simulink model "bpskRCdelayLG"  (Simulink 8.6)
settings: Solver=VariableStepAuto  StartTime=0.0  StopTime=10.0  RelTol=1e-3
values from neighbouring files (symbols this model uses):
  delay = .75    (= 0.75)    [lab02.m]    (also in setup.m = 0.5)
  filterspan = 4    [lab02.m]    (also in setup.m)
  outputSamples = 8    [lab02.m]    (also in setup.m)
  rolloff = .5    (= 0.5)    [lab02.m]    (also in setup.m)
  sampleTime = 1/R    (= 1.0272213662e-05)    [lab02.m]    (also in setup.m)
libraries: commdigbbndpm3 x2, commfilt2 x2, commchan3 x1, commsink2 x1, commsync2 x1, dspsigops x1
settings Model: Creator=tim  LastModifiedBy=tim
settings DataIOCC: SaveFormat=Dataset  SignalLoggingSaveFormat=Dataset
settings OptimizationCC: ExpressionDepthLimit=128
settings DebuggingCC: UnderspecifiedInitializationDetection=Simplified  MergeDetectMultiDrivingBlocksExec=error  SolverPrmCheckMsg=none  FcnCallInpInsideContextMsg=EnableAllAsError  StateNameClashWarn=none
settings HardwareCC: ProdBitPerPointer=64  ProdLargestAtomicFloat=Float  ProdIntDivRoundTo=Zero  ProdEndianess=LittleEndian  ProdWordSize=64  ProdHWDeviceType=Intel->x86-64 (Windows64)
settings GRTTargetCC: GeneratePreprocessorConditionals=Use local settings  CombineOutputUpdateFcns=on  GRTInterface=off
settings ConfigComp: CovModelRefEnable=off

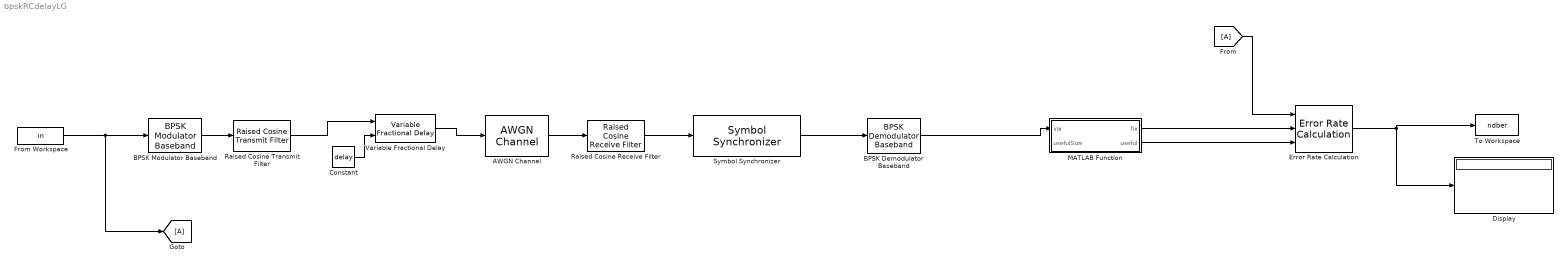
== system bpskRCdelayLG ==
  AWGN Channel : commchan3/AWGN Channel  InputProcessing=Columns as channels (frame based)  seed=67  noiseMode="Signal to noise ratio  (SNR)"  EbNodB=snr  EsNodB=10  SNRdB=snr  bitsPerSym=1  Ps=1  Tsym=1  variance=1
  BPSK Demodulator Baseband : commdigbbndpm3/BPSK Demodulator Baseband  Ph=0  DecType=Hard decision  VarSource=Dialog  Variance=1  outDtype=Inherit via internal rule  derotateFactorWordLen=16
  BPSK Modulator Baseband : commdigbbndpm3/BPSK Modulator Baseband  Ph=0  outDtype=double  outWordLen=16  outUDDataType=sfix(16)  outFracLenMode=Best precision  outFracLen=15
  Constant : Constant  Value=delay
  Display : Display
  Error Rate Calculation : commsink2/Error Rate Calculation  N=0  st_delay=0  cp_mode=Select samples from port  subframe=[]  PMode=Port  WsName=ErrorVec  RsMode2=off  stop=on  numErr=maxErrors  maxBits=maxBits
  From Workspace : FromWorkspace  VariableName=in  SampleTime=sampleTime  Interpolate=off  OutputAfterFinalValue=Cyclic repetition
  MATLAB Function : MATLAB Function  TreatAsAtomicUnit=on
  Raised Cosine Receive Filter : commfilt2/Raised Cosine Receive Filter  filtType=Square root  N=8  filtSpan=4  currentFiltSpan=4  D=(4)/2  R=.5  sampMode=Mute  saveAsFlag=0  rateMode=Downsampling  downFactor=1  downOffset=0  framing=Enforce single-rate processing  InputProcessing=Columns as channels (frame based)  checkGain=Normalized  filterGain=1  checkCoeff=off  variableName=rcRxFilt  launchFVT=on  roundingMode=Floor  overflowMode=off
  Raised Cosine Transmit Filter : commfilt2/Raised Cosine Transmit Filter  filtType=Square root  filtSpan=filterspan  currentFiltSpan=filterspan  D=(filterspan)/2  R=rolloff  sampMode=Mute  saveAsFlag=0  N=outputSamples  framing=Enforce single-rate processing  InputProcessing=Columns as channels (frame based)  checkGain=Normalized  filterGain=linearAmp  checkCoeff=off  variableName=rcTxFilt  launchFVT=on  roundingMode=Floor  overflowMode=off
  Symbol Synchronizer : commsync2/Symbol Synchronizer  TimingErrorDetector=Early-Late (non-data-aided)  SamplesPerSymbol=8  DampingFactor=1  NormalizedLoopBandwidth=.001  DetectorGain=2.7  TimingErrorOutputPort=off  SimulateUsing=Code generation
  To Workspace : ToWorkspace  VariableName=ndber  SampleTime=-1
      settings: Save2DSignal=2-D array (concatenate along first dimension)
  Variable Fractional Delay : dspsigops/Variable Fractional Delay  mode=OBSOLETE  modeActive=Linear  dmax=100  InputProcessing=Columns as channels (frame based)  L=4  FarrowL=4  R=10  alpha=1  ic=0  fallbackFIR=Clip to the minimum value necessary for centered kernel  fallbackFarrow=Clip to the minimum value necessary for centered kernel  noDFT=off  roundingMode=Zero  overflowMode=off
  wires:
  From Workspace/1 -> [A], BPSK Modulator Baseband/1
  Error Rate Calculation/1 -> To Workspace/1, Display/1
  BPSK Modulator Baseband/1 -> Raised Cosine Transmit Filter/1
  Raised Cosine Transmit Filter/1 -> Variable Fractional Delay/1
  AWGN Channel/1 -> Raised Cosine Receive Filter/1
  Variable Fractional Delay/1 -> AWGN Channel/1
  Constant/1 -> Variable Fractional Delay/2
  Raised Cosine Receive Filter/1 -> Symbol Synchronizer/1
  Symbol Synchronizer/1 -> BPSK Demodulator Baseband/1
  BPSK Demodulator Baseband/1 -> MATLAB Function/1(var)
  [A] -> Error Rate Calculation/1
  MATLAB Function/1(fix) -> Error Rate Calculation/2
  MATLAB Function/2(useful) -> Error Rate Calculation/3

== matlab function MATLAB Function ==
  data: var input double; fix output double size=[1000,1]; useful output double size=[1000,1]; usefulSize input double
function [fix,useful] = vartofix(var,usefulSize)
%#codegen
useful = zeros(1000,1);
fix = zeros(1000,1);
fix(1:usefulSize,1) = var;
useful((1:usefulSize),1) = ones(usefulSize,1);
end
